simulink model "stiffnessLPVModel"  (Simulink 8.7)
settings: Solver=ode3  StartTime=0.0  StopTime=simulationTime  FixedStep=simulationSamplingTime  RelTol=1e-3
values from neighbouring files (symbols this model uses):
  simulationSamplingTime = 0.001    [simLPV_ParallelCascade.m]    (also in simulate_LPV_ParallelCascade.m)
libraries: dsppolyfun x2
settings Model: Creator=Kian  LastModifiedBy=kian
settings DebuggingCC: SolverPrmCheckMsg=warning

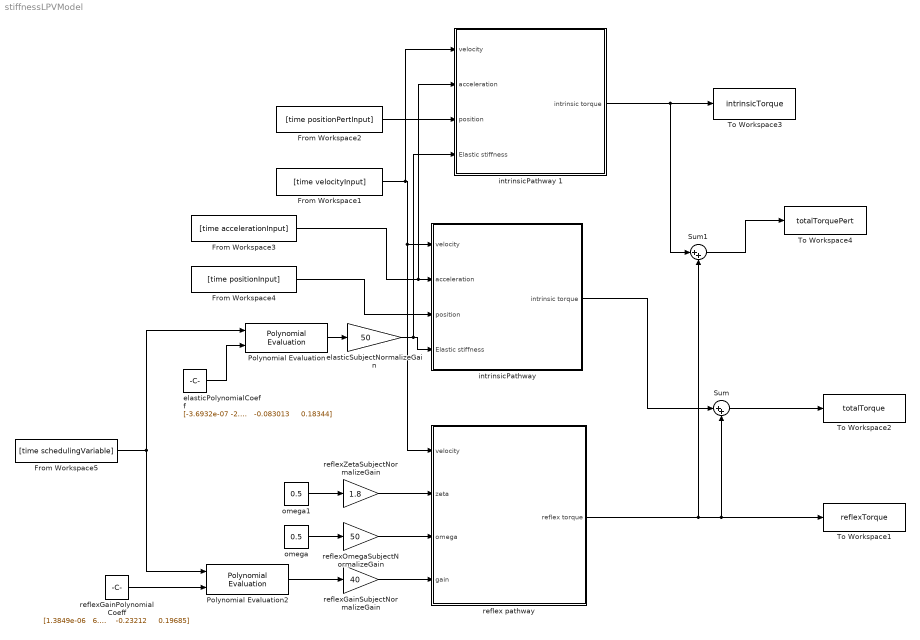
== system stiffnessLPVModel ==
  From Workspace1 : FromWorkspace  VariableName=[time velocityInput]  SampleTime=simulationSamplingTime
  From Workspace2 : FromWorkspace  VariableName=[time positionPertInput]  SampleTime=simulationSamplingTime
  From Workspace3 : FromWorkspace  VariableName=[time accelerationInput]  SampleTime=simulationSamplingTime
  From Workspace4 : FromWorkspace  VariableName=[time positionInput]  SampleTime=simulationSamplingTime
  From Workspace5 : FromWorkspace  VariableName=[time schedulingVariable]  SampleTime=simulationSamplingTime
  Polynomial Evaluation : dsppolyfun/Polynomial Evaluation  useConstCoeffs=off  constCoeffs=[5 4 3 2 1]
  Polynomial Evaluation2 : dsppolyfun/Polynomial Evaluation  useConstCoeffs=off  constCoeffs=[5 4 3 2 1]
  Sum : Sum  Inputs=|++
  Sum1 : Sum  Inputs=|++
  To Workspace1 : ToWorkspace  VariableName=reflexTorque  SampleTime=simulationSamplingTime
  To Workspace2 : ToWorkspace  VariableName=totalTorque  SampleTime=simulationSamplingTime
  To Workspace3 : ToWorkspace  VariableName=intrinsicTorque  SampleTime=simulationSamplingTime
  To Workspace4 : ToWorkspace  VariableName=totalTorquePert  SampleTime=simulationSamplingTime
  elasticPolynomialCoeff : Constant  Value="[-3.6932e-07 -2.2537e-05  -0.0005248  -0.0067572   -0.083013     0.18344]"
  elasticSubjectNormalizeGain : Gain  Gain=50
  "intrinsicPathway " : Subsystem
  intrinsicPathway 1 : Subsystem
  omega : Constant  Value=0.5
  omega1 : Constant  Value=0.5
  reflex pathway : Subsystem
  reflexGainPolynomialCoeff : Constant  Value="[1.3849e-06   6.439e-05  0.00031647   -0.019678    -0.23212     0.19685]"
  reflexGainSubjectNormalizeGain : Gain  Gain=40
  reflexOmegaSubjectNormalizeGain : Gain  Gain=50
  reflexZetaSubjectNormalizeGain : Gain  Gain=1.8
  wires:
  Polynomial Evaluation/1 -> elasticSubjectNormalizeGain/1
  elasticPolynomialCoeff/1 -> Polynomial Evaluation/2
  From Workspace5/1 -> Polynomial Evaluation2/1, Polynomial Evaluation/1
  omega1/1 -> reflexZetaSubjectNormalizeGain/1
  omega/1 -> reflexOmegaSubjectNormalizeGain/1
  reflexZetaSubjectNormalizeGain/1 -> reflex pathway/2(zeta)
  reflexOmegaSubjectNormalizeGain/1 -> reflex pathway/3(omega)
  reflexGainSubjectNormalizeGain/1 -> reflex pathway/4(gain)
  reflexGainPolynomialCoeff/1 -> Polynomial Evaluation2/2
  Polynomial Evaluation2/1 -> reflexGainSubjectNormalizeGain/1
  reflex pathway/1(reflex torque) -> Sum1/2, To Workspace1/1, Sum/2
  Sum/1 -> To Workspace2/1
  "intrinsicPathway "/1(intrinsic torque) -> Sum/1
  elasticSubjectNormalizeGain/1 -> intrinsicPathway 1/4(Elastic stiffness), "intrinsicPathway "/4(Elastic stiffness)
  From Workspace4/1 -> "intrinsicPathway "/3(position)
  From Workspace1/1 -> intrinsicPathway 1/1(velocity), "intrinsicPathway "/1(velocity), reflex pathway/1(velocity)
  From Workspace3/1 -> intrinsicPathway 1/2(acceleration), "intrinsicPathway "/2(acceleration)
  From Workspace2/1 -> intrinsicPathway 1/3(position)
  intrinsicPathway 1/1(intrinsic torque) -> Sum1/1, To Workspace3/1
  Sum1/1 -> To Workspace4/1

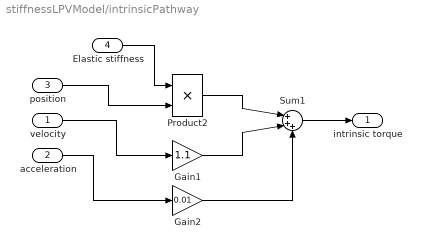
== system stiffnessLPVModel/intrinsicPathway  ==
  velocity : Inport
  acceleration : Inport  Port=2
  position : Inport  Port=3
  Elastic stiffness : Inport  Port=4
  Gain1 : Gain  Gain=1.1
  Gain2 : Gain  Gain=0.01
  Product2 : Product
  Sum1 : Sum  Inputs=|+++
  intrinsic torque : Outport
  wires:
  Elastic stiffness/1 -> Product2/1
  position/1 -> Product2/2
  velocity/1 -> Gain1/1
  acceleration/1 -> Gain2/1
  Product2/1 -> Sum1/1
  Gain1/1 -> Sum1/2
  Gain2/1 -> Sum1/3
  Sum1/1 -> intrinsic torque/1

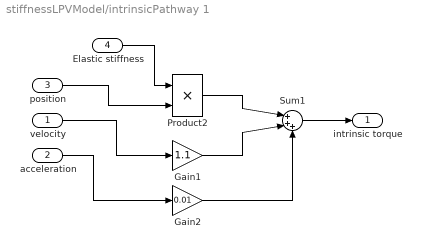
== system stiffnessLPVModel/intrinsicPathway 1 ==
  velocity : Inport
  acceleration : Inport  Port=2
  position : Inport  Port=3
  Elastic stiffness : Inport  Port=4
  Gain1 : Gain  Gain=1.1
  Gain2 : Gain  Gain=0.01
  Product2 : Product
  Sum1 : Sum  Inputs=|+++
  intrinsic torque : Outport
  wires:
  Elastic stiffness/1 -> Product2/1
  position/1 -> Product2/2
  velocity/1 -> Gain1/1
  acceleration/1 -> Gain2/1
  Product2/1 -> Sum1/1
  Gain1/1 -> Sum1/2
  Gain2/1 -> Sum1/3
  Sum1/1 -> intrinsic torque/1

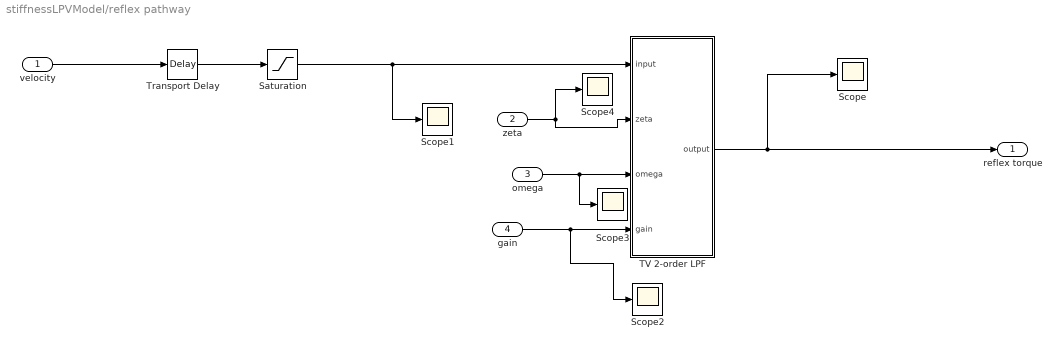
== system stiffnessLPVModel/reflex pathway ==
  velocity : Inport
  zeta : Inport  Port=2
  omega : Inport  Port=3
  gain : Inport  Port=4
  Saturation : Saturate  UpperLimit=Inf  LowerLimit=0
  Scope{,1..4} (5 alike) : Scope
  TV 2-order LPF : Subsystem
  Transport Delay : TransportDelay  DelayTime=0.05
  reflex torque : Outport
  wires:
  TV 2-order LPF/1(output) -> reflex torque/1, Scope/1
  velocity/1 -> Transport Delay/1
  Saturation/1 -> Scope1/1, TV 2-order LPF/1(input)
  Transport Delay/1 -> Saturation/1
  zeta/1 -> TV 2-order LPF/2(zeta), Scope4/1
  gain/1 -> Scope2/1, TV 2-order LPF/4(gain)
  omega/1 -> Scope3/1, TV 2-order LPF/3(omega)

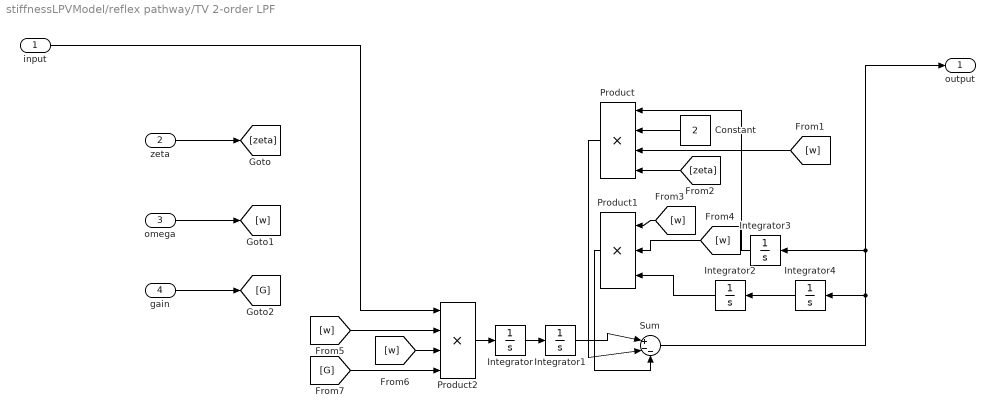
== system stiffnessLPVModel/reflex pathway/TV 2-order LPF ==
  input : Inport
  zeta : Inport  Port=2
  omega : Inport  Port=3
  gain : Inport  Port=4
  Constant : Constant  Value=2
  Integrator{,1..4} (5 alike) : Integrator
  Product : Product  Inputs=4
  Product1 : Product  Inputs=3
  Product2 : Product  Inputs=4
  Sum : Sum  Inputs=|+--
  output : Outport
  wires:
  Integrator1/1 -> Sum/1
  Integrator/1 -> Integrator1/1
  Product2/1 -> Integrator/1
  Integrator3/1 -> Product/1
  Integrator2/1 -> Product1/3
  Sum/1 -> Integrator4/1, output/1, Integrator3/1
  Integrator4/1 -> Integrator2/1
  input/1 -> Product2/1
  gain/1 -> [G]
  Product1/1 -> Sum/3
  [w] -> Product2/3
  [w] -> Product2/2
  Constant/1 -> Product/2
  [w] -> Product1/1
  Product/1 -> Sum/2
  [w] -> Product/3
  zeta/1 -> [zeta]
  [zeta] -> Product/4
  [w] -> Product1/2
  [G] -> Product2/4
  omega/1 -> [w]
